simulink model "Tractive_System_model"  (R2025b)
settings: Solver=ode15s  StartTime=0  StopTime=169.89  MaxStep=1e-3  RelTol=1e-3  AbsTol=1e-6
PreLoadFcn:
  | vehicleData
undefined symbols (not defined in the file): FL, FR, RL, RR, vehicle
libraries: batteryecm_lib x281, fl_lib x86, nesl_utility x54, ee_lib x16, sdl_lib x10, SimscapeFluids_lib x3, BatteryEstimators x2, simulink x1, slpidlib x1, autolibshared x1, eePmsmFieldOrientedControl x1
(part 26 of 26)

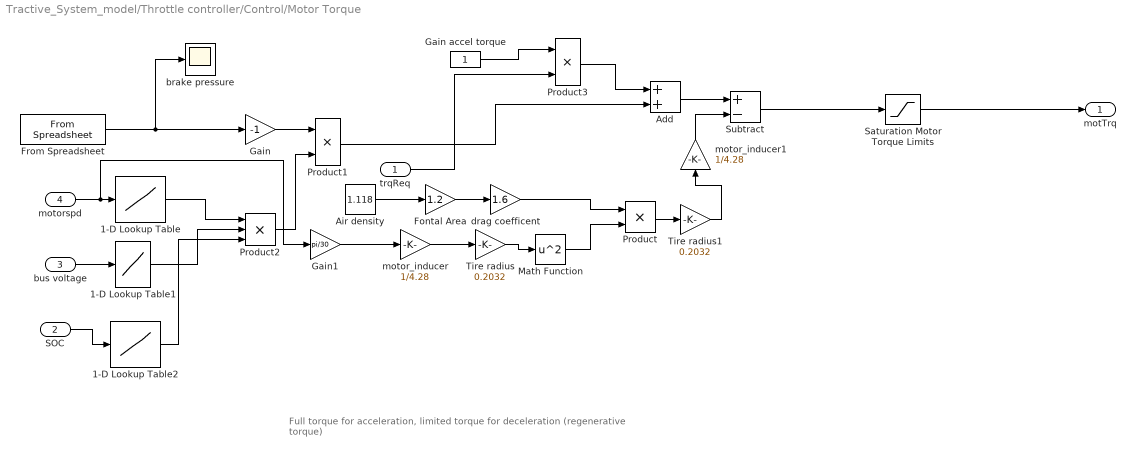
== system Tractive_System_model/Throttle controller/Control/Motor Torque ==
  note: Full torque for acceleration,
      | limited torque for deceleration (regenerative torque)
  trqReq : Inport
  SOC : Inport  Port=2
  bus voltage : Inport  Port=3
  motorspd : Inport  Port=4
  1-D Lookup Table : Lookup_n-D  NumberOfTableDimensions=1  BreakpointsForDimension1=[0,8,15,999]  Table=[0,0,1,1]  InternalRulePriority=Speed  RndMeth=Simplest
  1-D Lookup Table1 : Lookup_n-D  NumberOfTableDimensions=1  BreakpointsForDimension1=[0,540,560,999]  Table=[1,1,0,0]  InternalRulePriority=Speed  RndMeth=Simplest
  1-D Lookup Table2 : Lookup_n-D  NumberOfTableDimensions=1  BreakpointsForDimension1=[0,0.8,0.95,1]  Table=[1,1,0,0]  InternalRulePriority=Speed  RndMeth=Simplest
  Add : Sum
  Air density : Constant  Value=1.118
  Fontal Area : Gain  Gain=1.2
  From Spreadsheet : FromSpreadsheet  FileName=E25_Run1.xls  SheetName=Brake
  Gain : Gain  Gain=-1
  Gain accel torque : Constant
  Gain1 : Gain  Gain=pi/30
  Math Function : Math  Operator=square
  Product : Product
  Product1 : Product
  Product2 : Product  Inputs=3
  Product3 : Product
  Saturation Motor Torque Limits : Saturate  UpperLimit=150  LowerLimit=-150  ZeroCross=off
  Subtract : Sum  Inputs=+-
  Tire radius : Gain  Gain=0.2032
  Tire radius1 : Gain  Gain=0.2032
  brake pressure : Scope
      settings: ActiveDisplayYMinimum=-30.006488969158148  ActiveDisplayYMaximum=54.0625428368765  DataLoggingVariableName=ScopeData10
  drag coefficent : Gain  Gain=1.6
  motor_inducer : Gain  Gain=1/4.28
  motor_inducer1 : Gain  Gain=1/4.28
  motTrq : Outport
  wires:
  Saturation Motor Torque Limits/1 -> motTrq/1
  From Spreadsheet/1 -> brake pressure/1, Gain/1
  Gain/1 -> Product1/1
  SOC/1 -> 1-D Lookup Table2/1
  bus voltage/1 -> 1-D Lookup Table1/1
  1-D Lookup Table/1 -> Product2/1
  1-D Lookup Table1/1 -> Product2/2
  1-D Lookup Table2/1 -> Product2/3
  Product2/1 -> Product1/2
  Product1/1 -> Add/2
  Gain accel torque/1 -> Product3/1
  trqReq/1 -> Product3/2
  Product3/1 -> Add/1
  Add/1 -> Subtract/1
  Subtract/1 -> Saturation Motor Torque Limits/1
  Air density/1 -> Fontal Area/1
  Fontal Area/1 -> drag coefficent/1
  motorspd/1 -> Gain1/1, 1-D Lookup Table/1
  motor_inducer/1 -> Tire radius/1
  Tire radius/1 -> Math Function/1
  Math Function/1 -> Product/2
  drag coefficent/1 -> Product/1
  Tire radius1/1 -> motor_inducer1/1
  Product/1 -> Tire radius1/1
  motor_inducer1/1 -> Subtract/2
  Gain1/1 -> motor_inducer/1
